simulink model "ECM_opt_second"  (R2019b)
settings: Solver=ode4  StartTime=0  StopTime=max(Time_new)  FixedStep=0.05  RelTol=0.5e-4
values from neighbouring files (symbols this model uses):
  c1_opt = X(1)    [ECM_call_second.m]    (also in RCID_Single_Temp_Model_v3_mod.m = tau_1./ (r1_opt/1000))
  c2_opt = X(3)    [ECM_call_second.m]    (also in RCID_Single_Temp_Model_v3_mod.m = tau_2./ (r2_opt/1000))
  I_new = -1*I(Pulse_Start_Index(SOC_test)-5:Pulse_Start_Index(SOC_test)+Smallest_Pulse-1)    [RCID_Single_Temp_Model_old.m]    (also in RCID_Single_Temp_Model_v2.m; RCID_Single_Temp_Model_v3_mod.m = TestData.I(Pulse_Start_Index(i) : Pulse_Stop_Index(i)+300))
  ini_SOC_opt = SOC_count(Pulse_Start_Index(i))    [RCID_Single_Temp_Model_v3_mod.m]
  OCV = V(Initial_Pulse_Index)    [RCID_Single_Temp_Model_v3_mod.m]
  r1_opt = X(2)    [ECM_call_second.m]    (also in RCID_Single_Temp_Model_v3_mod.m = (abs(((TestData.V(Pulse_Start_Index(i) + 1) - TestData.V(Pul)
  r2_opt = X(4)    [ECM_call_second.m]    (also in RCID_Single_Temp_Model_v3_mod.m = (abs((TestData.V(Pulse_Start_Index(i) + R2_step) - TestData.)
  SOC = SOC_count(Initial_Pulse_Index)    [RCID_Single_Temp_Model_v3_mod.m]
  Time_new = Time(Pulse_Start_Index(SOC_test)-5:Pulse_Start_Index(SOC_test)+Smallest_Pulse-1)    [RCID_Single_Temp_Model_old.m]    (also in RCID_Single_Temp_Model_v2.m; RCID_Single_Temp_Model_v3_mod.m = TestData.Time(Pulse_Start_Index(i) : Pulse_Stop_Index(i)+300)
  V_new = V(Pulse_Start_Index(SOC_test)-5:Pulse_Start_Index(SOC_test)+Smallest_Pulse-1)    [RCID_Single_Temp_Model_old.m]    (also in RCID_Single_Temp_Model_v2.m; RCID_Single_Temp_Model_v3_mod.m = TestData.V(Pulse_Start_Index(i) : Pulse_Stop_Index(i)+300))
undefined symbols (not defined in the file or in its folder): r0_opt
settings Model: Creator=yatin  LastModifiedBy=yatin
settings DataIOCC: SaveFormat=Array  ReturnWorkspaceOutputs=off

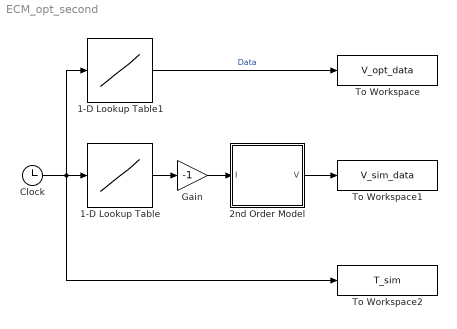
== system ECM_opt_second ==
  1-D Lookup Table : Lookup_n-D  NumberOfTableDimensions=1  BreakpointsForDimension1=Time_new  Table=I_new  InternalRulePriority=Speed  RndMeth=Simplest  InputSameDT=on
  1-D Lookup Table1 : Lookup_n-D  NumberOfTableDimensions=1  BreakpointsForDimension1=Time_new  Table=V_new  InternalRulePriority=Speed  RndMeth=Simplest  InputSameDT=on
  2nd Order Model : Subsystem
  Clock : Clock
  Gain : Gain  Gain=-1
  To Workspace : ToWorkspace  VariableName=V_opt_data  SampleTime=-1
  To Workspace1 : ToWorkspace  VariableName=V_sim_data  SampleTime=-1
  To Workspace2 : ToWorkspace  VariableName=T_sim  SampleTime=-1
  wires:
  1-D Lookup Table1/1 -> To Workspace/1  "Data"
  Clock/1 -> 1-D Lookup Table1/1, To Workspace2/1, 1-D Lookup Table/1
  2nd Order Model/1(V) -> To Workspace1/1
  1-D Lookup Table/1 -> Gain/1
  Gain/1 -> 2nd Order Model/1(I)

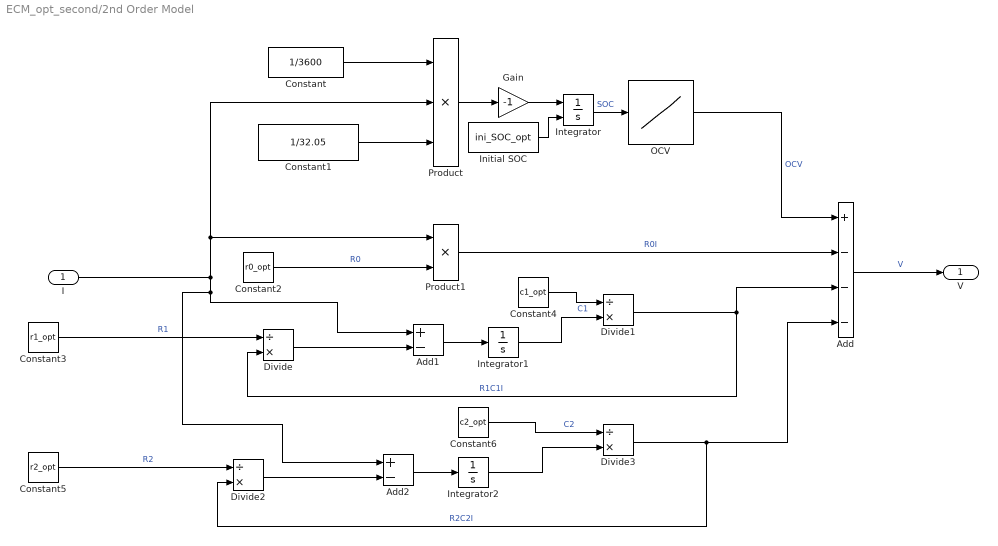
== system ECM_opt_second/2nd Order Model ==
  I : Inport
  Add : Sum  Inputs=+---
  Add1 : Sum  Inputs=+-
  Add2 : Sum  Inputs=+-
  Constant : Constant  Value=1/3600
  Constant1 : Constant  Value=1/32.05
  Constant2 : Constant  Value=r0_opt
  Constant3 : Constant  Value=r1_opt
  Constant4 : Constant  Value=c1_opt
  Constant5 : Constant  Value=r2_opt
  Constant6 : Constant  Value=c2_opt
  Divide{,1..3} (4 alike) : Product  Inputs=/*
  Gain : Gain  Gain=-1
  Initial SOC : Constant  Value=ini_SOC_opt
  Integrator : Integrator  InitialConditionSource=external
  Integrator1 : Integrator  UpperSaturationLimit=1  LowerSaturationLimit=0
  Integrator2 : Integrator  UpperSaturationLimit=1  LowerSaturationLimit=0
  OCV : Lookup_n-D  NumberOfTableDimensions=1  BreakpointsForDimension1=flip(SOC)  Table=flip(OCV)  InternalRulePriority=Speed  RndMeth=Simplest  InputSameDT=on
  Product : Product  Inputs=3
  Product1 : Product
  V : Outport
  wires:
  Initial SOC/1 -> Integrator/2
  Constant1/1 -> Product/3
  Product/1 -> Gain/1
  Integrator/1 -> OCV/1  "SOC"
  OCV/1 -> Add/1  "OCV"
  Add/1 -> V/1  "V"
  Product1/1 -> Add/2  "R0I"
  Constant/1 -> Product/1
  Constant2/1 -> Product1/2  "R0"
  Constant3/1 -> Divide/1  "R1"
  Divide/1 -> Add1/2
  Add1/1 -> Integrator1/1
  Integrator1/1 -> Divide1/2
  Constant4/1 -> Divide1/1  "C1"
  Divide1/1 -> Divide/2, Add/3  "R1C1I"
  Divide3/1 -> Add/4, Divide2/2  "R2C2I"
  Constant6/1 -> Divide3/1  "C2"
  I/1 -> Add2/1, Add1/1, Product/2, Product1/1
  Add2/1 -> Integrator2/1
  Integrator2/1 -> Divide3/2
  Divide2/1 -> Add2/2
  Constant5/1 -> Divide2/1  "R2"
  Gain/1 -> Integrator/1
